simulink model "Observer"  (R2022b)
settings: Solver=ode23t  StartTime=0.0  StopTime=15.0  MaxStep=0.01  MinStep=1e-7  RelTol=1e-6  AbsTol=1e-7
undefined symbols (not defined in the file or in its folder): A, A_obs, B, B_obs, C, C_obs, D, K_int, K_x
settings Model: Creator=emanuela  LastModifiedBy=emanuela
settings DataIOCC: SaveOutput=off  SignalLogging=off  DSMLogging=off  SaveTime=off  ReturnWorkspaceOutputs=off

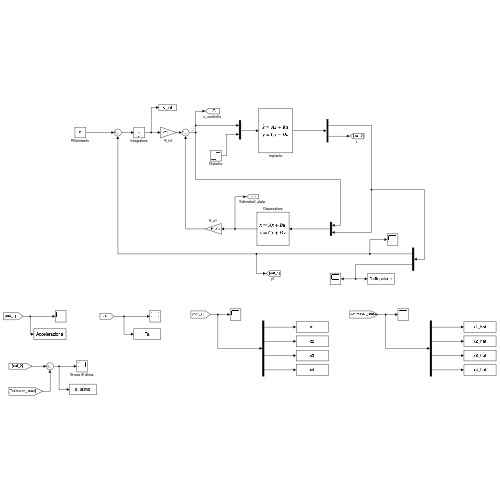
[thumbnail: Simulink's stored preview of the top-level diagram]
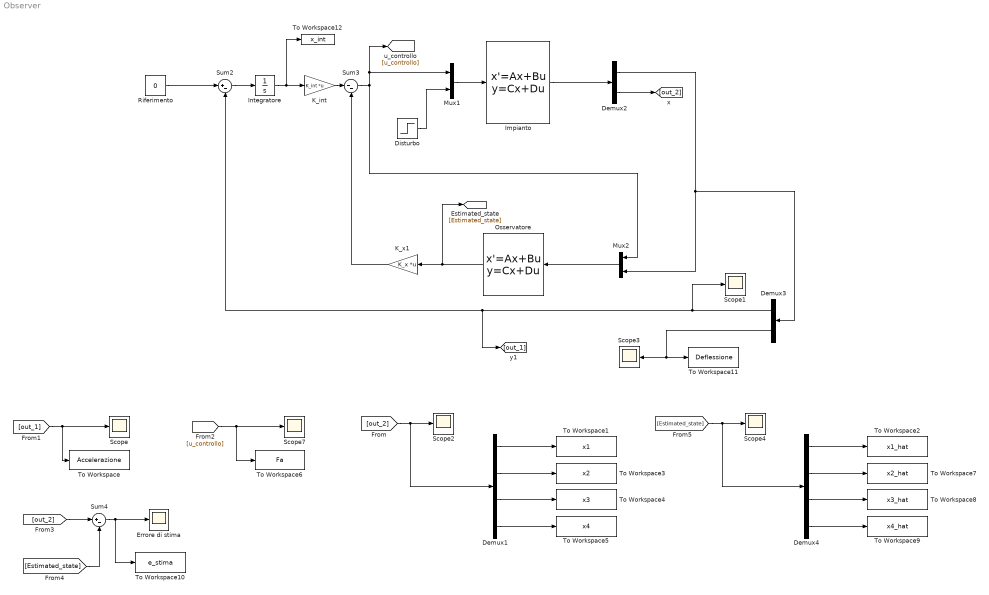
== system Observer ==
  Demux1 : Demux
  Demux2 : Demux  Outputs=[2,4]
  Demux3 : Demux  Outputs=2
  Demux4 : Demux
  Disturbo : Step  After=0.05  SampleTime=0
  Errore di stima : Scope
  Impianto : StateSpace  A=A  B=B  C=[C;eye(4)]  D=[D,;zeros(4,2)]  InitialCondition=0
  Integratore : Integrator
  K_int : Gain  Gain=K_int  Multiplication=Matrix(K*u)
  K_x1 : Gain  Gain=K_x  Multiplication=Matrix(K*u)
  Mux1 : Mux  Inputs=2
  Mux2 : Mux  Inputs=2
  Osservatore : StateSpace  A=A_obs  B=B_obs  C=C_obs  D=zeros(4,3)  InitialCondition=0 * ones(4,1);
  Riferimento : Constant  Value=0
  Scope{,1..4,7} (6 alike) : Scope
  Sum2 : Sum  Inputs=|+-
  Sum3 : Sum  Inputs=|--
  Sum4 : Sum  Inputs=|+-
  To Workspace : ToWorkspace  VariableName=Accelerazione  SaveFormat=Timeseries  SampleTime=-1
  To Workspace1 : ToWorkspace  VariableName=x1  SaveFormat=Timeseries  SampleTime=-1
  To Workspace10 : ToWorkspace  VariableName=e_stima  SaveFormat=Timeseries  SampleTime=-1
  To Workspace11 : ToWorkspace  VariableName=Deflessione  SaveFormat=Timeseries  SampleTime=-1
  To Workspace12 : ToWorkspace  VariableName=x_int  SaveFormat=Timeseries  SampleTime=-1
  To Workspace2 : ToWorkspace  VariableName=x1_hat  SaveFormat=Timeseries  SampleTime=-1
  To Workspace3 : ToWorkspace  VariableName=x2  SaveFormat=Timeseries  SampleTime=-1
  To Workspace4 : ToWorkspace  VariableName=x3  SaveFormat=Timeseries  SampleTime=-1
  To Workspace5 : ToWorkspace  VariableName=x4  SaveFormat=Timeseries  SampleTime=-1
  To Workspace6 : ToWorkspace  VariableName=Fa  SaveFormat=Timeseries  SampleTime=-1
  To Workspace7 : ToWorkspace  VariableName=x2_hat  SaveFormat=Timeseries  SampleTime=-1
  To Workspace8 : ToWorkspace  VariableName=x3_hat  SaveFormat=Timeseries  SampleTime=-1
  To Workspace9 : ToWorkspace  VariableName=x4_hat  SaveFormat=Timeseries  SampleTime=-1
  wires:
  [Estimated_state] -> Sum4/2
  Mux2/1 -> Osservatore/1
  Demux3/2 -> Scope3/1, To Workspace11/1
  Integratore/1 -> To Workspace12/1, K_int/1
  Sum2/1 -> Integratore/1
  Sum4/1 -> To Workspace10/1, Errore di stima/1
  K_x1/1 -> Sum3/2
  K_int/1 -> Sum3/1
  Riferimento/1 -> Sum2/1
  [out_2] -> Sum4/1
  Demux2/1 -> Mux2/2, Demux3/1
  Demux2/2 -> [out_2]
  Mux1/1 -> Impianto/1
  Impianto/1 -> Demux2/1
  Demux3/1 -> Scope1/1, [out_1], Sum2/2
  Osservatore/1 -> K_x1/1, [Estimated_state]
  Sum3/1 -> Mux2/1, Mux1/1, [u_controllo]
  [out_1] -> To Workspace/1, Scope/1
  [u_controllo] -> Scope7/1, To Workspace6/1
  [out_2] -> Demux1/1, Scope2/1
  Demux1/2 -> To Workspace3/1
  Demux1/4 -> To Workspace5/1
  Demux1/3 -> To Workspace4/1
  Demux1/1 -> To Workspace1/1
  Demux4/1 -> To Workspace2/1
  Demux4/3 -> To Workspace8/1
  Demux4/4 -> To Workspace9/1
  [Estimated_state] -> Demux4/1, Scope4/1
  Demux4/2 -> To Workspace7/1
  Disturbo/1 -> Mux1/2
